simulink model "closed_loop_freq_todo2"  (R2016b)
settings: Solver=VariableStepAuto  StartTime=0.0  StopTime=10.0  RelTol=1e-3
values from neighbouring files (symbols this model uses):
  delay_freq = 0.001    [LCSproject.m]
  test_den = cell2mat(test.Denominator)    [LCSproject.m]
  test_num = cell2mat(test.Numerator)    [LCSproject.m]
settings Model: Creator=Olivier  LastModifiedBy=Olivier

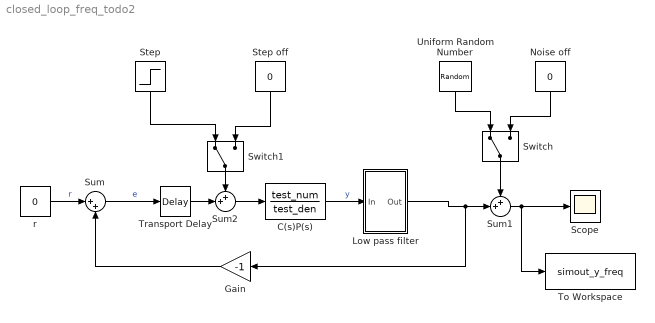
== system closed_loop_freq_todo2 ==
  C(s)P(s) : TransferFcn  Numerator=test_num  Denominator=test_den
  Gain : Gain  Gain=-1
  Low pass filter : Subsystem
  Noise off : Constant  Value=0
  Scope : Scope
  Step : Step  After=0.2  SampleTime=0
  Step off : Constant  Value=0
  Sum : Sum  Inputs=|++
  Sum1 : Sum  Inputs=++|
  Sum2 : Sum  Inputs=++|
  Switch : ManualSwitch
  Switch1 : ManualSwitch
  To Workspace : ToWorkspace  VariableName=simout_y_freq  SaveFormat=Timeseries  SampleTime=-1
  Transport Delay : TransportDelay  DelayTime=delay_freq
  Uniform Random Number : UniformRandomNumber  Minimum=-0.005  Maximum=0.005  SampleTime=0.1
  r : Constant  Value=0
  wires:
  r/1 -> Sum/1  "r"
  Uniform Random Number/1 -> Switch/1
  Gain/1 -> Sum/2
  Transport Delay/1 -> Sum2/2
  Sum1/1 -> To Workspace/1, Scope/1
  Sum2/1 -> C(s)P(s)/1
  Step/1 -> Switch1/1
  Sum/1 -> Transport Delay/1  "e"
  Noise off/1 -> Switch/2
  Switch/1 -> Sum1/1
  Switch1/1 -> Sum2/1
  Step off/1 -> Switch1/2
  C(s)P(s)/1 -> Low pass filter/1(In)  "y"
  Low pass filter/1(Out) -> Gain/1, Sum1/2

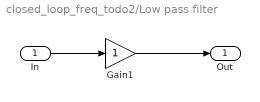
== system closed_loop_freq_todo2/Low pass filter ==
  In : Inport
  Gain1 : Gain
  Out : Outport
  wires:
  In/1 -> Gain1/1
  Gain1/1 -> Out/1
